simulink model "flightControlSystem"  (R2024b)
settings: Solver=ode3  StartTime=0  StopTime=TFinal  FixedStep=Ts  RelTol=1e-3  EnableMultiTasking=on
undefined symbols (not defined in the file): codertarget, Controller, DiscIntNeverNeededParam, Discrete, Estimator, g, init, Sensors, Time, Ts, var_acc_angle_N, var_bias_gyr_N, var_gyro_p_N, Vehicle
libraries: simulink x37, slpidlib x4, ctrlSharedLib x4, sharedtransform x3, visionanalysis x1, visiontransforms x1, parrotlib x1
(part 3 of 3)

== stateflow chart flightControlSystem/Control System/Path Planning/Chart ==
  state NavigateTrack
    state North
      entry:
      current = "N";
      isAtEnd = false;
      during:
      xout = xout + 0.0005;
      isAtEnd = isEndOfDirection(directions, "N", threshold);
    state NorthEast
      entry:
      current = "NE";
      isAtEnd = false;
      during:
      xout = xout + 0.0005;
      yout = yout + 0.0005;
      isAtEnd = isEndOfDirection(directions, "NE", threshold);
    state Find_Direction_
      entry:
      [direction, threshold] = findDirection(directions, current);
      xout = xout;
      yout = yout;
      zout = zout;
    NorthEast -> Find_Direction_ : [isAtEnd == true]
    North -> Find_Direction_ : [isAtEnd == true]
    Find_Direction_ -> North [order 1] : [direction == "N"]
    Find_Direction_ -> NorthEast [order 2] : [direction == "NE"]
    (default) -> Find_Direction_
  state Land_
    state SoftLanding
      entry:
      current = "Landing";
      during:
      zout = zout + 0.0005;
    state centersAroundCircle [commented out]
    (default) -> SoftLanding
  state Takeoff
    entry:
    xout = 0;
    yout = 0;
    zout = -1.1;
  state Hover [commented out]
    entry:
    xout = 0;
    yout = 0;
    zout = -1.1;
  state MoveForward [commented out]
    during:
    xout = 1.3;
    yout = 0;
    zout = -1.1;
  state MoveRight [commented out]
    during:
    xout = 2.5;
    yout = 1.2;
    zout = -1.1;
  state MoveFinal [commented out]
    during:
    xout = 3.7;
    yout = 1.2;
    zout = -1.1;
  state Land [commented out]
    during:
    xout = 4;
    yout = 1.3;
    zout = 0;
  (default) -> Takeoff
  Takeoff -> NavigateTrack : [after(5, sec)]
  NavigateTrack -> Land_ : [after(50,sec)]
  (default) -> Hover [commented out]
  Hover -> MoveForward [commented out] : [after(5, sec)]
  MoveForward -> MoveRight [commented out] : [after(8, sec)]
  MoveRight -> MoveFinal [commented out] : [after(8, sec)]
  MoveFinal -> Land [commented out] : [after(8, sec)]
  data: directionVector function_input; currentDir function_input; curDirection function_output; curThreshold function_output; directionVector function_input; currentDir function_input; hasReachedEnd function_output; curThreshold function_input; xout output double; yout output double; zout output double; directions input uint32; direction local string; current local string ="Start"; isAtEnd local boolean =false; threshold local uint32
  function [curDirection, curThreshold] = findDirection(directionVector, currentDir):
    | function [curDirection, curThreshold] = findDirection(directionVector, currentDir)
    | 
    | curDirection = "N";
    | curThreshold = directionVector(1);
    | 
    | if currentDir == "N"
    |     if directionVector(5) > directionVector(6)
    |         curDirection = "NE";
    |         curThreshold = directionVector(5);
    |     else
    |         curDirection = "NW";
    |         curThreshold = directionVector(6);
    |     end
    | elseif currentDir == "E"
    |     if directionVector(5) > directionVector(7)
    |         curDirection = "NE";
    |         curThreshold = directionVector(5);
    |     else
    |         curDirection = "SE";
    |         curThreshold = directionVector(7);
    |     end
    | elseif currentDir == "S"
    |     if directionVector(7) > directionVector(8)
    |         curDirection = "SE";
    |         curThreshold = directionVector(7);
    |     else
    |         curDirection = "SW";
    |         curThreshold = directionVector(8);
    |     end
    | elseif currentDir == "W"
    |     if directionVector(6) > directionVector(8)
    |         curDirection = "NW";
    |     else
    |         curDirection = "SW";
    |     end
    | elseif currentDir == "NE"
    |     if directionVector(1) > directionVector(2)
    |         curDirection = "N";
    |         curThreshold = directionVector(1);
    |     else
    |         curDirection = "E";
    |         curThreshold = directionVector(2);
    |     end
    | elseif currentDir == "NW"
    |     if directionVector(1) > directionVector(4)
    |         curDirection = "N";
    |         curThreshold = directionVector(1);
    |     else
    |         curDirection = "W";
    |         curThreshold = directionVector(4);
    |     end
    | elseif currentDir == "SE"
    |     if directionVector(3) > directionVector(2)
    |         curDirection = "S";
    |         curThreshold = directionVector(3);
    |     else
    |         curDirection = "E";
    |         curThreshold = directionVector(2);
    |     end
    | elseif currentDir == "SW"
    |     if directionVector(3) > directionVector(4)
    |         curDirection = "S";
    |         curThreshold = directionVector(3);
    |     else
    |         curDirection = "W";
    |         curThreshold = directionVector(4);
    |     end
    | % else
    | %     [~, index] = max(directionVector);
    | %     if index == 1
    | %         curDirection = "N";
    | %         curThreshold = directionVector(1);
    | %     elseif index == 2
    | %         curDirection = "E";
    | %         curThreshold = directionVector(2);
    | %     elseif index == 3
    | %         curDirection = "S";
    | %         curThreshold = directionVector(3);
    | %     elseif index == 4
    | %         curDirection = "W";
    | %         curThreshold = directionVector(4);
    | %     elseif index == 5
    | %         curDirection = "NE";
    | %         curThreshold = directionVector(5);
    | %     elseif index == 6
    | %         curDirection = "NW";
    | %         curThreshold = directionVector(6);
    | %     elseif index == 7
    | %         curDirection = "SE";
    | %         curThreshold = directionVector(7);
    | %     elseif index == 8
    | %         curDirection = "SW";
    | %         curThreshold = directionVector(8);
    | %     else
    | %         curDirection = "N";
    | %         curThreshold = directionVector(1);
    | %     end
    | end
  function hasReachedEnd = isEndOfDirection(directionVector, currentDir, curThreshold):
    | function hasReachedEnd = isEndOfDirection(directionVector, currentDir, curThreshold)
    | 
    | if currentDir == "N"
    |     index = 1;
    | elseif currentDir == "E"
    |     index = 2;
    | elseif currentDir == "S"
    |     index = 3;
    | elseif currentDir == "W"
    |     index = 4;
    | elseif currentDir == "NE"
    |     index = 5;
    | elseif currentDir == "NW"
    |     index = 6;
    | elseif currentDir == "SE"
    |     index = 7;
    | elseif currentDir == "SW"
    |     index = 8;
    | end
    | 
    | if directionVector(index) < ((80/100) * curThreshold)
    |     hasReachedEnd = true;
    | else
    |     hasReachedEnd = false;
    | end
  function centerAroundCircle:
    | function centerAroundCircle
